simulink model "sampleModel208"  (R2021b)
settings: Solver=VariableStepAuto  StartTime=0.0  StopTime=10.0  RelTol=1e-3
undefined symbols (not defined in the file or in its folder): DiscIntNeverNeededParam, Newton, Raphson
libraries: simulink x23, slpidlib x3
settings Model: Creator=user  LastModifiedBy=user

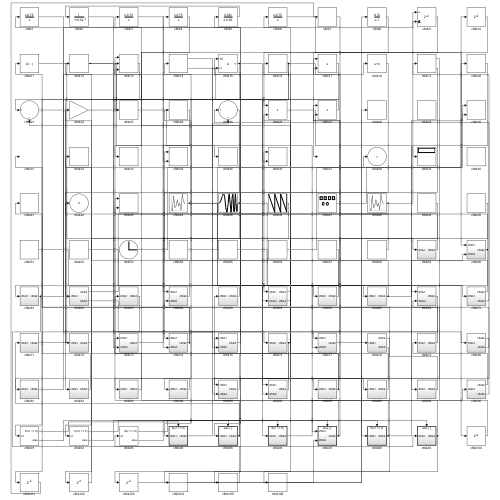
[thumbnail: Simulink's stored preview of the top-level diagram]
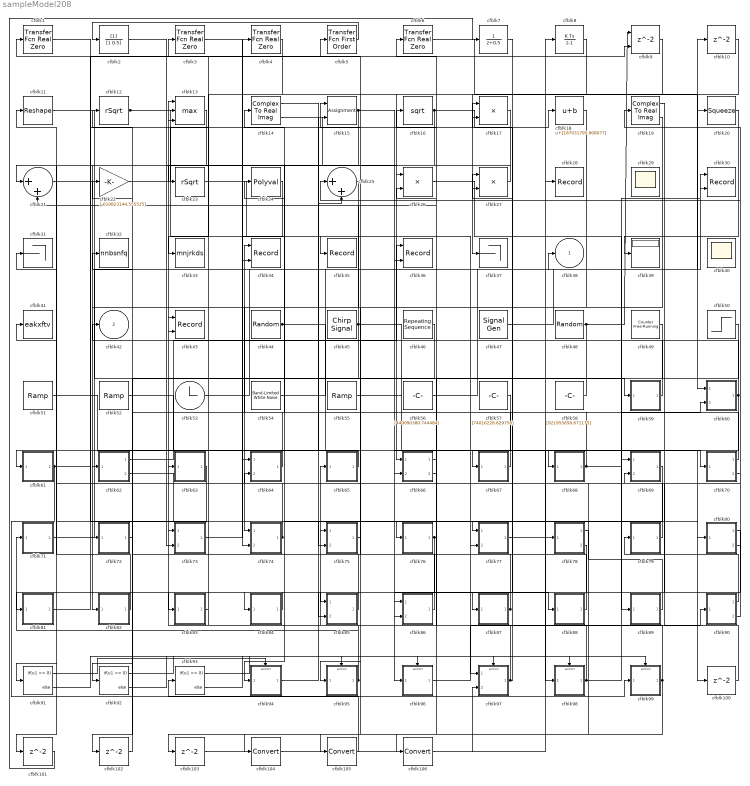
== system sampleModel208 ==
  cfblk{1,3..4,6} (4 alike) : simulink/Discrete/Transfer Fcn Real Zero  ZeroZ=0.75  ICPrevInput=0.0  DoSatur=off
      settings: SourceProductBaseCode=SL
  cfblk{10,100..103} (5 alike) : Delay  SampleTime=1
  cfblk104 : DataTypeConversion
  cfblk105 : DataTypeConversion
  cfblk106 : DataTypeConversion
  cfblk11 : Reshape
  cfblk12 : Sqrt  Operator=rSqrt  AlgorithmType=Newton-Raphson  SaturateOnIntegerOverflow=on
  cfblk13 : MinMax  Function=max  Inputs=3
  cfblk14 : ComplexToRealImag
  cfblk15 : Assignment  DiagnosticForDimensions=Warning  IndexOptions=Index vector (dialog)  Indices=1  OutputSizes=1
  cfblk16 : Sqrt  SaturateOnIntegerOverflow=on
  cfblk17 : Product
  cfblk18 : Bias  Bias=[187031795.908077]
  cfblk19 : ComplexToRealImag
  cfblk2 : DiscreteFilter  SampleTime=1
  cfblk20 : Squeeze
  cfblk21 : Sum  Inputs=|++
  cfblk22 : Gain  Gain=[-610823144.555525]
  cfblk23 : Sqrt  Operator=rSqrt  AlgorithmType=Newton-Raphson  SaturateOnIntegerOverflow=on
  cfblk24 : Polyval  Coefs=[ +2.081618890e-019, -1.441693666e-014, +4.719686976e-010, -8.536869453e-006, +1.621573104e-001, -8.087801117e+001 ]
  cfblk25 : Sum  Inputs=|++
  cfblk26 : Product
  cfblk27 : Product  Inputs=**
  cfblk28 : Record  FileSettingsInternal="{\"entries\":[{\"content\":{\"excelSettings\":{\"content\":{},\"type\":\"Streamout.ExcelSettings\"}},\"type\":\"Streamout.FileSettingStorage\",\"uuid\":\"c22ba1ce-0fcd-43a5-9d90-0db8329606c8\"}],\"packageUris\":[\"http://schema.mathworks.com/mf0/streamout_blocks/R2020a\"],\"version\":\"1.0\"}"  SignalsInternal="{\"entries\":[{\"content\":{\"signals\":[{\"content\":{\"blockPath\":[\"sampleModel208/cfblk28\"],\"channel\":[],\"dimensions\":[1],\"domain\":\"sampleModel208/cfblk28\",\"lineColor\":\"#d95319\",\"plots\":[1],\"port\":1,\"sid\":[\"\"],\"signalID\":8022,\"signalName\":\"cfblk104\"},\"type\":\"RecordBlkView.Signal\",\"uuid\":\"261dbd1d-26c2-4045-9e24-154e5f0ad3fe\"}]},\"type\":\"RecordBlkView.InputSignals\",\"uuid\":\"b79c4309-7b5a-40c4-895f-b2cc34602c3d\"}],\"packageUris\":[\"http://schema.mathworks.com/mf0/streamout_blocks/R2020a\"],\"version\":\"1.0\"}"  VisualizationBindings="{\"sparklinesplugin\":{\"info\":[{\"bindingParametersList\":[],\"subplotID\":1}]}}"
  cfblk29 : Scope
      settings: Floating=on
  cfblk30 : Record  FileSettingsInternal="{\"entries\":[{\"content\":{\"excelSettings\":{\"content\":{},\"type\":\"Streamout.ExcelSettings\"}},\"type\":\"Streamout.FileSettingStorage\",\"uuid\":\"b5dc1131-858a-47e8-ba90-4585db02b6d4\"}],\"packageUris\":[\"http://schema.mathworks.com/mf0/streamout_blocks/R2020a\"],\"version\":\"1.0\"}"  Layout=[1 1]  SignalsInternal="{\"entries\":[{\"content\":{\"signals\":[{\"content\":{\"blockPath\":[\"sampleModel208/cfblk30\"],\"channel\":[],\"dimensions\":[1],\"domain\":\"sampleModel208/cfblk30\",\"lineColor\":\"#a2142f\",\"plots\":[1],\"port\":1,\"sid\":[\"\"],\"signalID\":8026,\"signalName\":\"cfblk54\"},\"type\":\"RecordBlkView.Signal\",\"uuid\":\"3317f2e0-9c09-47a8-be30-a309801c78f4\"},{\"content\":{\"blockPath\":[\"sampleModel208/cfblk30\"],\"channel\":[],\"dimensions\":[1],\"domain\":\"sampleModel208/cfblk30\",\"lineColor\":\"#139fff\",\"plots\":[1],\"port\":2,\"sid\":[\"\"],\"signalID\":8030,\"signalName\":\"cfblk68\"},\"type\":\"RecordBlkView.Signal\",\"uuid\":\"8cfe8237-c0e8-4d48-b3ed-0524deef0457\"}]},\"type\":\"RecordBlkView.InputSignals\",\"uuid\":\"ba5baa30-43f7-4293-854a-121f9ae80c9b\"}],\"packageUris\":[\"http://schema.mathworks.com/mf0/streamout_blocks/R2020a\"],\"version\":\"1.0\"}"  VisualizationBindings="{\"xyplotplugin\":{\"info\":[{\"series\":[{\"bindingParametersList\":[{\"parameter\":\"X-Axis\",\"signalID\":8026,\"signalName\":\"cfblk54\"},{\"parameter\":\"Y-Axis\",\"signalID\":8030,\"signalName\":\"cfblk68\"}],\"seriesID\":18668}],\"subplotID\":1}]}}"  CompatibilityTag=XY
  cfblk31 : Terminator
  cfblk32 : ToWorkspace  VariableName=nnbsnfq  SaveFormat=Timeseries  SampleTime=-1
  cfblk33 : ToWorkspace  VariableName=mnjrkds  SaveFormat=Timeseries  SampleTime=-1
  cfblk34 : Record  FileSettingsInternal="{\"entries\":[{\"content\":{\"excelSettings\":{\"content\":{},\"type\":\"Streamout.ExcelSettings\"}},\"type\":\"Streamout.FileSettingStorage\",\"uuid\":\"4f32d4e9-02ed-4236-9ce3-c0bcdef04756\"}],\"packageUris\":[\"http://schema.mathworks.com/mf0/streamout_blocks/R2020a\"],\"version\":\"1.0\"}"  Layout=[1 1]  SignalsInternal="{\"entries\":[{\"content\":{\"signals\":[{\"content\":{\"blockPath\":[\"sampleModel208/cfblk34\"],\"channel\":[],\"dimensions\":[1],\"domain\":\"sampleModel208/cfblk34\",\"lineColor\":\"#a2142f\",\"plots\":[1],\"port\":1,\"sid\":[\"\"],\"signalID\":8054,\"signalName\":\"cfblk64\"},\"type\":\"RecordBlkView.Signal\",\"uuid\":\"7ea00e73-cf0b-4523-9dfb-d0665cf2003d\"},{\"content\":{\"blockPath\":[\"sampleModel208/cfblk34\"],\"channel\":[],\"dimensions\":[1],\"domain\":\"sampleModel208/cfblk34\",\"lineColor\":\"#139fff\",\"plots\":[1],\"port\":2,\"sid\":[\"\"],\"signalID\":8058,\"signalName\":\"cfblk24\"},\"type\":\"RecordBlkView.Signal\",\"uuid\":\"3ec3da29-cb72-43d4-ab85-a156e7dbbd36\"}]},\"type\":\"RecordBlkView.InputSignals\",\"uuid\":\"b859cf70-4a05-42e5-becb-aa8dfd0be4f3\"}],\"packageUris\":[\"http://schema.mathworks.com/mf0/streamout_blocks/R2020a\"],\"version\":\"1.0\"}"  VisualizationBindings="{\"xyplotplugin\":{\"info\":[{\"series\":[{\"bindingParametersList\":[{\"parameter\":\"X-Axis\",\"signalID\":8054,\"signalName\":\"cfblk64\"},{\"parameter\":\"Y-Axis\",\"signalID\":8058,\"signalName\":\"cfblk24\"}],\"seriesID\":28405}],\"subplotID\":1}]}}"  CompatibilityTag=XY
  cfblk35 : Record  FileSettingsInternal="{\"entries\":[{\"content\":{\"excelSettings\":{\"content\":{},\"type\":\"Streamout.ExcelSettings\"}},\"type\":\"Streamout.FileSettingStorage\",\"uuid\":\"4d5d1943-00c1-4ccc-bfc5-894631c5acb5\"}],\"packageUris\":[\"http://schema.mathworks.com/mf0/streamout_blocks/R2020a\"],\"version\":\"1.0\"}"  SignalsInternal="{\"entries\":[{\"content\":{\"signals\":[{\"content\":{\"blockPath\":[\"sampleModel208/cfblk35\"],\"channel\":[],\"dimensions\":[1],\"domain\":\"sampleModel208/cfblk35\",\"lineColor\":\"#77ac30\",\"plots\":[1],\"port\":1,\"sid\":[\"\"],\"signalID\":8034,\"signalName\":\"cfblk23\"},\"type\":\"RecordBlkView.Signal\",\"uuid\":\"a308330b-7e8f-4a04-a4b5-6eaafb41392d\"}]},\"type\":\"RecordBlkView.InputSignals\",\"uuid\":\"e134a712-f80f-465f-b2ee-20551d8e1273\"}],\"packageUris\":[\"http://schema.mathworks.com/mf0/streamout_blocks/R2020a\"],\"version\":\"1.0\"}"  VisualizationBindings="{\"sparklinesplugin\":{\"info\":[{\"bindingParametersList\":[],\"subplotID\":1}]}}"
  cfblk36 : Record  FileSettingsInternal="{\"entries\":[{\"content\":{\"excelSettings\":{\"content\":{},\"type\":\"Streamout.ExcelSettings\"}},\"type\":\"Streamout.FileSettingStorage\",\"uuid\":\"a0d14922-92c5-4109-8193-fc27ce21709e\"}],\"packageUris\":[\"http://schema.mathworks.com/mf0/streamout_blocks/R2020a\"],\"version\":\"1.0\"}"  Layout=[1 1]  SignalsInternal="{\"entries\":[{\"content\":{\"signals\":[{\"content\":{\"blockPath\":[\"sampleModel208/cfblk36\"],\"channel\":[],\"dimensions\":[1],\"domain\":\"sampleModel208/cfblk36\",\"lineColor\":\"#a2142f\",\"plots\":[1],\"port\":1,\"sid\":[\"\"],\"signalID\":8038,\"signalName\":\"cfblk62:1\"},\"type\":\"RecordBlkView.Signal\",\"uuid\":\"cf392b0d-73b1-445c-b980-8f3ea822809a\"},{\"content\":{\"blockPath\":[\"sampleModel208/cfblk36\"],\"channel\":[],\"dimensions\":[1],\"domain\":\"sampleModel208/cfblk36\",\"lineColor\":\"#139fff\",\"plots\":[1],\"port\":2,\"sid\":[\"\"],\"signalID\":8042,\"signalName\":\"cfblk16\"},\"type\":\"RecordBlkView.Signal\",\"uuid\":\"24cc8bd0-c2dc-4a3d-a0ab-d3c31cd0a1be\"}]},\"type\":\"RecordBlkView.InputSignals\",\"uuid\":\"8c2f2ea3-48ed-4664-b571-c4b9f4e82adb\"}],\"packageUris\":[\"http://schema.mathworks.com/mf0/streamout_blocks/R2020a\"],\"version\":\"1.0\"}"  VisualizationBindings="{\"xyplotplugin\":{\"info\":[{\"series\":[{\"bindingParametersList\":[{\"parameter\":\"X-Axis\",\"signalID\":8038,\"signalName\":\"cfblk62:1\"},{\"parameter\":\"Y-Axis\",\"signalID\":8042,\"signalName\":\"cfblk16\"}],\"seriesID\":24383}],\"subplotID\":1}]}}"  CompatibilityTag=XY
  cfblk37 : Terminator
  cfblk39 : Display
  cfblk40 : Scope
      settings: Floating=on
  cfblk41 : ToWorkspace  VariableName=eakxftv  SaveFormat=Timeseries  SampleTime=-1
  cfblk43 : Record  FileSettingsInternal="{\"entries\":[{\"content\":{\"excelSettings\":{\"content\":{},\"type\":\"Streamout.ExcelSettings\"}},\"type\":\"Streamout.FileSettingStorage\",\"uuid\":\"00404128-d092-4654-98f3-0c769e6ce3be\"}],\"packageUris\":[\"http://schema.mathworks.com/mf0/streamout_blocks/R2020a\"],\"version\":\"1.0\"}"  Layout=[1 1]  SignalsInternal="{\"entries\":[{\"content\":{\"signals\":[{\"content\":{\"blockPath\":[\"sampleModel208/cfblk43\"],\"channel\":[],\"dimensions\":[1],\"domain\":\"sampleModel208/cfblk43\",\"lineColor\":\"#a2142f\",\"plots\":[1],\"port\":1,\"sid\":[\"\"],\"signalID\":8046,\"signalName\":\"cfblk79\"},\"type\":\"RecordBlkView.Signal\",\"uuid\":\"ce2b062f-3cfe-4973-a794-e20ce7e23f9b\"},{\"content\":{\"blockPath\":[\"sampleModel208/cfblk43\"],\"channel\":[],\"dimensions\":[1],\"domain\":\"sampleModel208/cfblk43\",\"lineColor\":\"#139fff\",\"plots\":[1],\"port\":2,\"sid\":[\"\"],\"signalID\":8050,\"signalName\":\"cfblk48\"},\"type\":\"RecordBlkView.Signal\",\"uuid\":\"da814807-78ce-423b-937a-9547f0faf18a\"}]},\"type\":\"RecordBlkView.InputSignals\",\"uuid\":\"e4b74333-ca83-42be-81e0-1eb5d34b8ec7\"}],\"packageUris\":[\"http://schema.mathworks.com/mf0/streamout_blocks/R2020a\"],\"version\":\"1.0\"}"  VisualizationBindings="{\"xyplotplugin\":{\"info\":[{\"series\":[{\"bindingParametersList\":[{\"parameter\":\"X-Axis\",\"signalID\":8046,\"signalName\":\"cfblk79\"},{\"parameter\":\"Y-Axis\",\"signalID\":8050,\"signalName\":\"cfblk48\"}],\"seriesID\":25686}],\"subplotID\":1}]}}"  CompatibilityTag=XY
  cfblk44 : UniformRandomNumber  Minimum=[-5209162267.996864]  Maximum=[7486341106.977611]  Seed=[64925626.000000]  SampleTime=0.1
  cfblk45 : simulink/Sources/Chirp Signal  f1=[-755698620.571404]  T=[-833933526.641706]  f2=[267223703.943291]
  cfblk46 : simulink/Sources/Repeating Sequence  rep_seq_t=[0 2]  rep_seq_y=[919874426.508816, 363568850.149377]
  cfblk47 : SignalGenerator  WaveForm=square  Amplitude=[217272616.194499]
  cfblk48 : UniformRandomNumber  Minimum=[-5223909817.198769]  Maximum=[5188022340.697088]  Seed=[56413417.000000]  SampleTime=0.1
  cfblk49 : simulink/Sources/Counter Free-Running  NumBits=[41.000000]  tsamp=-1
  cfblk5 : simulink/Discrete/Transfer Fcn First Order  PoleZ=0.95  ICPrevOutput=0.0  DoSatur=off
  cfblk50 : Step  Time=[15.000000]  Before=[292405392.362123]  After=[-377924494.241017]  SampleTime=0
  cfblk51 : simulink/Sources/Ramp  slope=[5467.724857]  start=[19.133778]  InitialOutput=[29297.594376]
  cfblk52 : simulink/Sources/Ramp  slope=[706.412132]  start=[13.023382]  InitialOutput=[-774712.176920]
  cfblk53 : Clock
  cfblk54 : simulink/Sources/Band-Limited White Noise  Cov=[6259669263.783980]  Ts=0.1  seed=[9291998557.000000]
  cfblk55 : simulink/Sources/Ramp  slope=[-6341.235505]  start=[31.577316]  InitialOutput=[-676904.104674]
  cfblk56 : Constant  Value=[440090380.744484]  SampleTime=1
  cfblk57 : Constant  Value=[74016228.829758]  SampleTime=1
  cfblk58 : Constant  Value=[921955858.671175]  SampleTime=1
  cfblk59 : Subsystem
  cfblk60 : Subsystem
  cfblk61 : Subsystem
  cfblk62 : Subsystem
  cfblk63 : Subsystem
  cfblk64 : Subsystem
  cfblk65 : Subsystem
  cfblk66 : Subsystem
  cfblk67 : Subsystem
  cfblk68 : Subsystem
  cfblk69 : Subsystem
  cfblk7 : DiscreteTransferFcn  SampleTime=1
  cfblk70 : Subsystem
  cfblk71 : Subsystem
  cfblk72 : Subsystem
  cfblk73 : Subsystem
  cfblk74 : Subsystem
  cfblk75 : Subsystem
  cfblk76 : Subsystem
  cfblk77 : Subsystem
  cfblk78 : Subsystem
  cfblk79 : Subsystem
  cfblk8 : DiscreteIntegrator  ICPrevOutput=DiscIntNeverNeededParam  ICPrevScaledInput=DiscIntNeverNeededParam
  cfblk80 : Subsystem
  cfblk81 : Subsystem
  cfblk82 : Subsystem
  cfblk83 : Subsystem
  cfblk84 : Subsystem
  cfblk85 : Subsystem
  cfblk86 : Subsystem
  cfblk87 : Subsystem
  cfblk88 : Subsystem
  cfblk89 : Subsystem
  cfblk9 : Delay  ShowEnablePort=on  SampleTime=1
      settings: InputPortMap=u0,e6
  cfblk90 : Subsystem
  cfblk91 : If  IfExpression=u1 >= 0  SampleTime=1
  cfblk92 : If  IfExpression=u1 >= 0  SampleTime=1
  cfblk93 : If  IfExpression=u1 >= 0  SampleTime=1
  cfblk94 : Subsystem  TreatAsAtomicUnit=on
  cfblk95 : Subsystem  TreatAsAtomicUnit=on
  cfblk96 : Subsystem  TreatAsAtomicUnit=on
  cfblk97 : Subsystem  TreatAsAtomicUnit=on
  cfblk98 : Subsystem  TreatAsAtomicUnit=on
  cfblk99 : Subsystem  TreatAsAtomicUnit=on
  cfblk38 : Outport
  cfblk42 : Outport  Port=2
  wires:
  cfblk64/1(cfblk2) -> cfblk34/1
  cfblk97/1(cfblk2) -> cfblk65/1(cfblk1), cfblk27/2
  cfblk88/1(cfblk2) -> cfblk75/1(cfblk1)
  cfblk9/1 -> cfblk66/1(cfblk1)
  cfblk90/1(cfblk2) -> cfblk79/1(cfblk1)
  cfblk13/1 -> cfblk82/1(cfblk1)
  cfblk89/1(cfblk2) -> cfblk1/1
  cfblk73/1(cfblk2) -> cfblk4/1
  cfblk95/1(cfblk2) -> cfblk71/1(cfblk1), cfblk73/1(cfblk1)
  cfblk16/1 -> cfblk18/1, cfblk36/2, cfblk73/2(cfblk5)
  cfblk58/1 -> cfblk14/1
  cfblk85/1(cfblk2) -> cfblk13/1
  cfblk90/2(cfblk5) -> cfblk25/1
  cfblk54/1 -> cfblk30/1
  cfblk10/1 -> cfblk37/1
  cfblk87/1(cfblk2) -> cfblk15/1, cfblk26/2
  cfblk61/1(cfblk2) -> cfblk99/1(cfblk1), cfblk13/3
  cfblk56/1 -> cfblk20/1
  cfblk18/1 -> cfblk95/1(cfblk1)
  cfblk83/1(cfblk2) -> cfblk3/1
  cfblk48/1 -> cfblk9/1, cfblk43/2
  cfblk65/1(cfblk2) -> cfblk61/1(cfblk1)
  cfblk23/1 -> cfblk35/1
  cfblk8/1 -> cfblk33/1
  cfblk12/1 -> cfblk97/1(cfblk1), cfblk76/1(cfblk1)
  cfblk51/1 -> cfblk68/1(cfblk1)
  cfblk27/1 -> cfblk21/1
  cfblk74/1(cfblk2) -> cfblk31/1, cfblk41/1
  cfblk79/1(cfblk2) -> cfblk43/1
  cfblk98/1(cfblk2) -> cfblk16/1, cfblk60/2(cfblk5)
  cfblk7/1 -> cfblk87/1(cfblk1)
  cfblk14/1 -> cfblk70/1(cfblk1)
  cfblk2/1 -> cfblk26/1
  cfblk71/1(cfblk2) -> cfblk38/1
  cfblk19/1 -> cfblk85/1(cfblk1)
  cfblk99/1(cfblk2) -> cfblk63/1(cfblk1), cfblk103/1
  cfblk84/1(cfblk2) -> cfblk81/1(cfblk1)
  cfblk52/1 -> cfblk80/1(cfblk1)
  cfblk81/1(cfblk2) -> cfblk9/2
  cfblk67/1(cfblk2) -> cfblk24/1
  cfblk82/1(cfblk2) -> cfblk11/1
  cfblk20/1 -> cfblk39/1
  cfblk19/2 -> cfblk74/1(cfblk1)
  cfblk44/1 -> cfblk89/1(cfblk1), cfblk96/1(cfblk1)
  cfblk75/1(cfblk2) -> cfblk5/1
  cfblk14/2 -> cfblk86/1(cfblk1)
  cfblk22/1 -> cfblk17/1
  cfblk94/1(cfblk2) -> cfblk25/2
  cfblk96/1(cfblk2) -> cfblk90/1(cfblk1)
  cfblk3/1 -> cfblk64/1(cfblk1)
  cfblk11/1 -> cfblk59/1(cfblk1)
  cfblk80/1(cfblk2) -> cfblk83/1(cfblk1)
  cfblk25/1 -> cfblk72/1(cfblk1)
  cfblk47/1 -> cfblk10/1
  cfblk5/1 -> cfblk2/1
  cfblk53/1 -> cfblk15/2
  cfblk24/1 -> cfblk34/2
  cfblk21/1 -> cfblk62/1(cfblk1)
  cfblk45/1 -> cfblk74/2(cfblk3), cfblk77/2(cfblk5), cfblk13/2
  cfblk6/1 -> cfblk60/1(cfblk1)
  cfblk76/1(cfblk2) -> cfblk6/1, cfblk86/2(cfblk5)
  cfblk63/1(cfblk2) -> cfblk91/1
  cfblk86/1(cfblk2) -> cfblk32/1
  cfblk55/1 -> cfblk98/1(cfblk1)
  cfblk66/1(cfblk2) -> cfblk85/2(cfblk4)
  cfblk15/1 -> cfblk88/1(cfblk1), cfblk101/1
  cfblk80/2(cfblk4) -> cfblk64/2(cfblk5)
  cfblk26/1 -> cfblk69/1(cfblk1)
  cfblk66/2(cfblk4) -> cfblk21/2
  cfblk77/1(cfblk2) -> cfblk8/1
  cfblk60/1(cfblk2) -> cfblk27/1, cfblk66/2(cfblk3)
  cfblk62/1(cfblk2) -> cfblk36/1
  cfblk59/1(cfblk2) -> cfblk42/1
  cfblk4/1 -> cfblk23/1
  cfblk17/1 -> cfblk94/1(cfblk1)
  cfblk46/1 -> cfblk92/1
  cfblk1/1 -> cfblk75/2(cfblk5)
  cfblk69/1(cfblk2) -> cfblk84/1(cfblk1)
  cfblk70/1(cfblk2) -> cfblk22/1
  cfblk57/1 -> cfblk67/1(cfblk1)
  cfblk70/2(cfblk3) -> cfblk19/1
  cfblk68/1(cfblk2) -> cfblk30/2, cfblk17/2
  cfblk50/1 -> cfblk77/1(cfblk1)
  cfblk91/1 -> cfblk94/Action
  cfblk91/2 -> cfblk95/Action
  cfblk92/1 -> cfblk96/Action
  cfblk92/2 -> cfblk97/Action
  cfblk93/1 -> cfblk98/Action
  cfblk93/2 -> cfblk99/Action
  cfblk62/2(cfblk3) -> cfblk100/1
  cfblk100/1 -> cfblk69/2(cfblk3)
  cfblk101/1 -> cfblk7/1
  cfblk72/1(cfblk2) -> cfblk102/1
  cfblk102/1 -> cfblk12/1
  cfblk103/1 -> cfblk97/2(cfblk4)
  cfblk78/1(cfblk2) -> cfblk104/1
  cfblk104/1 -> cfblk28/1
  cfblk78/2(cfblk3) -> cfblk105/1
  cfblk105/1 -> cfblk93/1
  cfblk49/1 -> cfblk106/1
  cfblk106/1 -> cfblk78/1(cfblk1)

== system sampleModel208/cfblk59 ==
  cfblk1 : Inport
  cfblk3 : DiscreteIntegrator  ICPrevOutput=DiscIntNeverNeededParam  ICPrevScaledInput=DiscIntNeverNeededParam
  cfblk2 : Outport
  wires:
  cfblk1/1 -> cfblk2/1, cfblk3/1

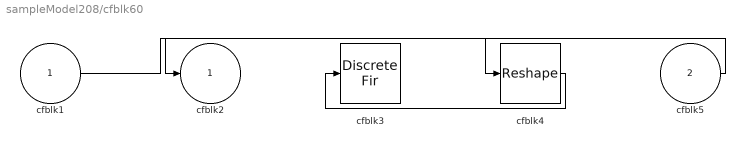
== system sampleModel208/cfblk60 ==
  cfblk1 : Inport
  cfblk5 : Inport  Port=2
  cfblk3 : DiscreteFir  SampleTime=1
  cfblk4 : Reshape
  cfblk2 : Outport
  wires:
  cfblk5/1 -> cfblk2/1
  cfblk4/1 -> cfblk3/1
  cfblk1/1 -> cfblk4/1

== system sampleModel208/cfblk61 ==
  cfblk1 : Inport
  cfblk3 : simulink/Discrete/Difference  ICPrevInput=0.0  OutMin=[]  OutMax=[]  OutDataTypeStr=Inherit: Inherit via back propagation  OutDataType=fixdt(1, 16)  OutScaling=2^-10  DoSatur=off
  cfblk4 : ComplexToRealImag
  cfblk2 : Outport
  wires:
  cfblk1/1 -> cfblk3/1
  cfblk4/1 -> cfblk2/1
  cfblk3/1 -> cfblk4/1

== system sampleModel208/cfblk62 ==
  cfblk1 : Inport
  cfblk2 : Outport
  cfblk3 : Outport  Port=2
  wires:
  cfblk1/1 -> cfblk2/1, cfblk3/1

== system sampleModel208/cfblk63 ==
  cfblk1 : Inport
  cfblk3 : Polyval  Coefs=[ +2.081618890e-019, -1.441693666e-014, +4.719686976e-010, -8.536869453e-006, +1.621573104e-001, -8.087801117e+001 ]
  cfblk2 : Outport
  wires:
  cfblk1/1 -> cfblk3/1
  cfblk3/1 -> cfblk2/1

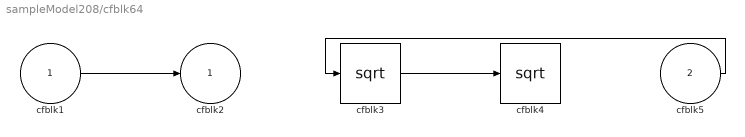
== system sampleModel208/cfblk64 ==
  cfblk1 : Inport
  cfblk5 : Inport  Port=2
  cfblk3 : Sqrt  SaturateOnIntegerOverflow=on
  cfblk4 : Sqrt  SaturateOnIntegerOverflow=on
  cfblk2 : Outport
  wires:
  cfblk1/1 -> cfblk2/1
  cfblk5/1 -> cfblk3/1
  cfblk3/1 -> cfblk4/1

== system sampleModel208/cfblk65 ==
  cfblk1 : Inport
  cfblk3 : Constant  Value=[606104915.024978]  SampleTime=1
  cfblk2 : Outport
  wires:
  cfblk1/1 -> cfblk2/1

== system sampleModel208/cfblk66 ==
  cfblk1 : Inport
  cfblk3 : Inport  Port=2
  cfblk2 : Outport
  cfblk4 : Outport  Port=2
  wires:
  cfblk3/1 -> cfblk4/1
  cfblk1/1 -> cfblk2/1

== system sampleModel208/cfblk67 ==
  cfblk1 : Inport
  cfblk3 : Delay  SampleTime=1
  cfblk4 : slpidlib/PID Controller  Controller=PID  Form=Parallel  TimeDomain=Discrete-time  UseExternalTs=off  SampleTime=1  IntegratorMethod=Forward Euler  FilterMethod=Forward Euler  ControllerParametersSource=internal  P=1  I=1  D=0  UseFilter=on  N=100  TunerSelectOption=Transfer Function Based (PID Tuner App)  InitialConditionSource=internal  InitialConditionForIntegrator=0  InitialConditionForFilter=0  DifferentiatorICPrevScaledInput=0  ExternalReset=none  TrackingMode=off  Kt=1  LimitOutput=off  SatLimitsSource=internal  UpperSaturationLimit=inf  LowerSaturationLimit=-inf  LinearizeAsGain=off  AntiWindupMode=none  Kb=1  POutMin=[]  POutMax=[]  IOutMin=[]  IOutMax=[]  DOutMin=[]  DOutMax=[]  NOutMin=[]  NOutMax=[]  SumOutMin=[]  SumOutMax=[]  SaturationOutMin=[]  SaturationOutMax=[]  PParamMin=[]  PParamMax=[]  IParamMin=[]  IParamMax=[]  DParamMin=[]  DParamMax=[]  NParamMin=[]  NParamMax=[]  KbParamMin=[]  KbParamMax=[]  KtParamMin=[]  KtParamMax=[]  KbOutMin=[]  KbOutMax=[]  KtOutMin=[]  KtOutMax=[]  IntegratorOutMin=[]  IntegratorOutMax=[]  FilterOutMin=[]  FilterOutMax=[]  SumI1OutMin=[]  SumI1OutMax=[]  SumI2OutMin=[]  SumI2OutMax=[]  SumI3OutMin=[]  SumI3OutMax=[]  SumI4OutMin=[]  SumI4OutMax=[]  SumDOutMin=[]  SumDOutMax=[]  DifferentiatorOutMin=[]  DifferentiatorOutMax=[]  FilterDiffOutCoefMin=[]  FilterDiffOutCoefMax=[]  ReciprocalOutMin=[]  ReciprocalOutMax=[]  SumDenOutMin=[]  SumDenOutMax=[]  SumNumOutMin=[]  SumNumOutMax=[]  DivideOutMin=[]  DivideOutMax=[]  UdiffTsProdOutMin=[]  UdiffTsProdOutMax=[]  NTsProdOutMin=[]  NTsProdOutMax=[]  UintegralTsProdOutMin=[]  UintegralTsProdOutMax=[]  UngainTsProdOutMin=[]  UngainTsProdOutMax=[]  IntegratorContinuousStateAttributes=''  IntegratorStateMustResolveToSignalObject=off  IntegratorRTWStateStorageClass=Auto  FilterContinuousStateAttributes=''  FilterStateMustResolveToSignalObject=off  FilterRTWStateStorageClass=Auto  ParallelPVariant=InternalParameters  IdealPVariant=Disabled  IVariant=InternalParameters  DVariant=InternalParameters  IntegratorVariant=Discrete  SatVariant=Disabled  AWVariant=Passthrough  PCopyVariant=Disabled  TRVariant=Disabled  FdbkBlocksVariant=Forward  IdealPFdbkVariant=Disabled  SatFdbkVariant=Disabled  DerivativeFilterVariant=ForwardEulerFilter  NVariant=InternalParameters  NCopyVariant=Disabled  FilterICVariant=InternalICsFilter  IntegratorICVariant=InternalICs  ExternalResetVariant=Disabled  TRSumVariant=Passthrough  SumFdbkVariant=Disabled  SumVariant=Sum_PID  TsampFilterVariant=InternalTs  TsampNgainVariant=Passthrough  TsampIntegralVariant=Passthrough  ExternalSaturationOutDataTypeStr=Inherit: Same as second input
  cfblk2 : Outport
  wires:
  cfblk1/1 -> cfblk3/1
  cfblk4/1 -> cfblk2/1
  cfblk3/1 -> cfblk4/1

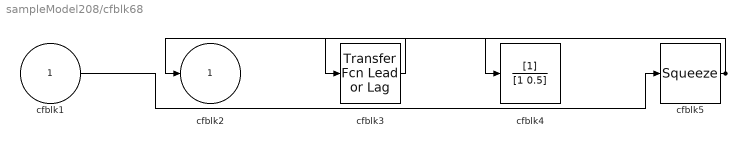
== system sampleModel208/cfblk68 ==
  cfblk1 : Inport
  cfblk3 : simulink/Discrete/Transfer Fcn Lead or Lag  PoleZ=0.95  ZeroZ=0.75  ICPrevOutput=0.0  ICPrevInput=0.0  DoSatur=off
      settings: SourceProductBaseCode=SL
  cfblk4 : DiscreteFilter  SampleTime=1
  cfblk5 : Squeeze
  cfblk2 : Outport
  wires:
  cfblk3/1 -> cfblk2/1
  cfblk1/1 -> cfblk5/1
  cfblk5/1 -> cfblk3/1, cfblk4/1

== system sampleModel208/cfblk69 ==
  cfblk1 : Inport
  cfblk3 : Inport  Port=2
  cfblk2 : Outport
  wires:
  cfblk1/1 -> cfblk2/1

== system sampleModel208/cfblk70 ==
  cfblk1 : Inport
  cfblk2 : Outport
  cfblk3 : Outport  Port=2
  wires:
  cfblk1/1 -> cfblk3/1, cfblk2/1

== system sampleModel208/cfblk71 ==
  cfblk1 : Inport
  cfblk3 : Math  Operator=conj  SaturateOnIntegerOverflow=on
  cfblk2 : Outport
  wires:
  cfblk3/1 -> cfblk2/1
  cfblk1/1 -> cfblk3/1

== system sampleModel208/cfblk72 ==
  cfblk1 : Inport
  cfblk3 : Delay  ShowEnablePort=on  SampleTime=1
      settings: InputPortMap=u0,e6
  cfblk2 : Outport
  wires:
  cfblk3/1 -> cfblk2/1
  cfblk1/1 -> cfblk3/1, cfblk3/2

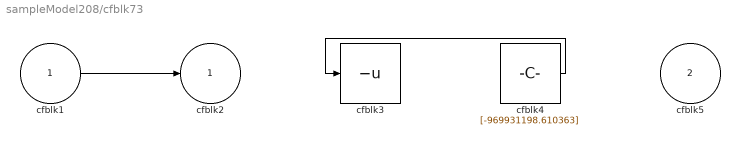
== system sampleModel208/cfblk73 ==
  cfblk1 : Inport
  cfblk5 : Inport  Port=2
  cfblk3 : UnaryMinus
  cfblk4 : Constant  Value=[-969931198.610363]  SampleTime=1
  cfblk2 : Outport
  wires:
  cfblk1/1 -> cfblk2/1
  cfblk4/1 -> cfblk3/1

== system sampleModel208/cfblk74 ==
  cfblk1 : Inport
  cfblk3 : Inport  Port=2
  cfblk2 : Outport
  wires:
  cfblk3/1 -> cfblk2/1

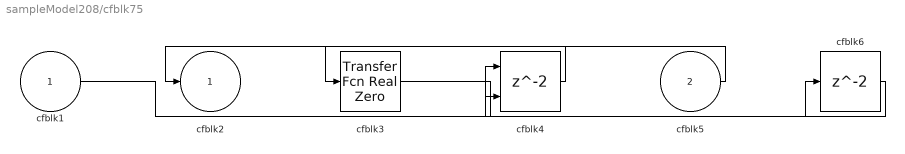
== system sampleModel208/cfblk75 ==
  cfblk1 : Inport
  cfblk5 : Inport  Port=2
  cfblk3 : simulink/Discrete/Transfer Fcn Real Zero  ZeroZ=0.75  ICPrevInput=0.0  DoSatur=off
      settings: SourceProductBaseCode=SL
  cfblk4 : Delay  ShowEnablePort=on  SampleTime=1
      settings: InputPortMap=u0,e6
  cfblk6 : Delay  SampleTime=1
  cfblk2 : Outport
  wires:
  cfblk5/1 -> cfblk2/1
  cfblk1/1 -> cfblk4/1
  cfblk4/1 -> cfblk3/1
  cfblk3/1 -> cfblk6/1
  cfblk6/1 -> cfblk4/2

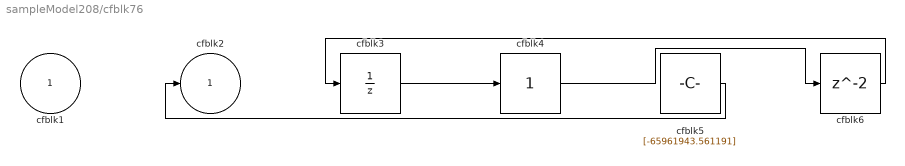
== system sampleModel208/cfblk76 ==
  cfblk1 : Inport
  cfblk3 : UnitDelay  HasFrameUpgradeWarning=on
  cfblk4 : simulink/Math Operations/Slider Gain  gain=1  low=0  high=2
  cfblk5 : Constant  Value=[-65961943.561191]  SampleTime=1
  cfblk6 : Delay  SampleTime=1
  cfblk2 : Outport
  wires:
  cfblk3/1 -> cfblk4/1
  cfblk5/1 -> cfblk2/1
  cfblk4/1 -> cfblk6/1
  cfblk6/1 -> cfblk3/1

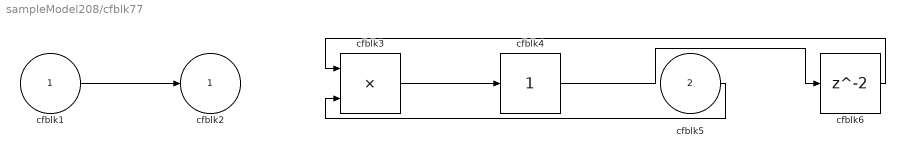
== system sampleModel208/cfblk77 ==
  cfblk1 : Inport
  cfblk5 : Inport  Port=2
  cfblk3 : Product
  cfblk4 : simulink/Math Operations/Slider Gain  gain=1  low=0  high=2
  cfblk6 : Delay  SampleTime=1
  cfblk2 : Outport
  wires:
  cfblk1/1 -> cfblk2/1
  cfblk3/1 -> cfblk4/1
  cfblk5/1 -> cfblk3/2
  cfblk4/1 -> cfblk6/1
  cfblk6/1 -> cfblk3/1

== system sampleModel208/cfblk78 ==
  cfblk1 : Inport
  cfblk2 : Outport
  cfblk3 : Outport  Port=2
  wires:
  cfblk1/1 -> cfblk2/1, cfblk3/1

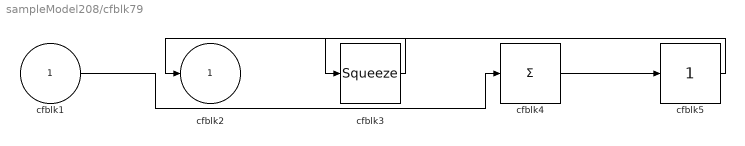
== system sampleModel208/cfblk79 ==
  cfblk1 : Inport
  cfblk3 : Squeeze
  cfblk4 : Sum  Inputs=+
  cfblk5 : simulink/Math Operations/Slider Gain  gain=1  low=0  high=2
  cfblk2 : Outport
  wires:
  cfblk4/1 -> cfblk5/1
  cfblk3/1 -> cfblk2/1
  cfblk1/1 -> cfblk4/1
  cfblk5/1 -> cfblk3/1

== system sampleModel208/cfblk80 ==
  cfblk1 : Inport
  cfblk3 : Constant  Value=[142919699.194080]  SampleTime=1
  cfblk2 : Outport
  cfblk4 : Outport  Port=2
  wires:
  cfblk1/1 -> cfblk2/1
  cfblk3/1 -> cfblk4/1

== system sampleModel208/cfblk81 ==
  cfblk1 : Inport
  cfblk3 : Sum  Inputs=|++
  cfblk2 : Outport
  wires:
  cfblk1/1 -> cfblk3/1, cfblk3/2
  cfblk3/1 -> cfblk2/1

== system sampleModel208/cfblk82 ==
  cfblk1 : Inport
  cfblk3 : Product  Inputs=**
  cfblk2 : Outport
  wires:
  cfblk1/1 -> cfblk3/1, cfblk3/2
  cfblk3/1 -> cfblk2/1

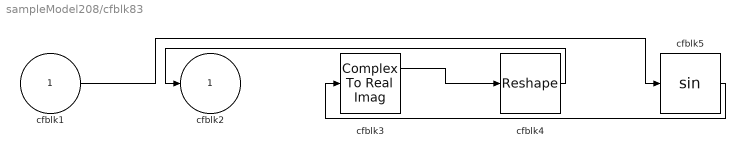
== system sampleModel208/cfblk83 ==
  cfblk1 : Inport
  cfblk3 : ComplexToRealImag
  cfblk4 : Reshape
  cfblk5 : Trigonometry
  cfblk2 : Outport
  wires:
  cfblk4/1 -> cfblk2/1
  cfblk5/1 -> cfblk3/1
  cfblk1/1 -> cfblk5/1
  cfblk3/1 -> cfblk4/1

== system sampleModel208/cfblk84 ==
  cfblk1 : Inport
  cfblk3 : simulink/Discrete/Difference  ICPrevInput=0.0  OutMin=[]  OutMax=[]  OutDataTypeStr=Inherit: Inherit via back propagation  OutDataType=fixdt(1, 16)  OutScaling=2^-10  DoSatur=off
  cfblk4 : Reshape
  cfblk2 : Outport
  wires:
  cfblk1/1 -> cfblk4/1
  cfblk4/1 -> cfblk3/1
  cfblk3/1 -> cfblk2/1

== system sampleModel208/cfblk85 ==
  cfblk1 : Inport
  cfblk4 : Inport  Port=2
  cfblk3 : Constant  Value=[587237413.607553]  SampleTime=1
  cfblk2 : Outport
  wires:
  cfblk3/1 -> cfblk2/1

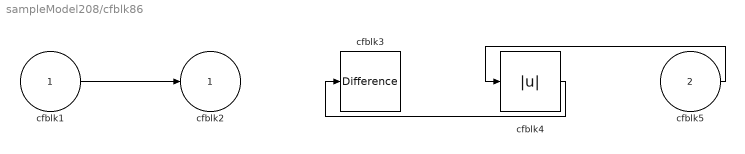
== system sampleModel208/cfblk86 ==
  cfblk1 : Inport
  cfblk5 : Inport  Port=2
  cfblk3 : simulink/Discrete/Difference  ICPrevInput=0.0  OutMin=[]  OutMax=[]  OutDataTypeStr=Inherit: Inherit via back propagation  OutDataType=fixdt(1, 16)  OutScaling=2^-10  DoSatur=off
  cfblk4 : Abs
  cfblk2 : Outport
  wires:
  cfblk1/1 -> cfblk2/1
  cfblk5/1 -> cfblk4/1
  cfblk4/1 -> cfblk3/1

== system sampleModel208/cfblk87 ==
  cfblk1 : Inport
  cfblk3 : simulink/Discrete/Transfer Fcn Real Zero  ZeroZ=0.75  ICPrevInput=0.0  DoSatur=off
      settings: SourceProductBaseCode=SL
  cfblk2 : Outport
  wires:
  cfblk1/1 -> cfblk3/1
  cfblk3/1 -> cfblk2/1

== system sampleModel208/cfblk88 ==
  cfblk1 : Inport
  cfblk3 : ComplexToMagnitudeAngle
  cfblk4 : Sin  TimeSource=Use external signal  SampleTime=0
  cfblk2 : Outport
  wires:
  cfblk4/1 -> cfblk3/1
  cfblk1/1 -> cfblk4/1
  cfblk3/1 -> cfblk2/1

== system sampleModel208/cfblk89 ==
  cfblk1 : Inport
  cfblk3 : slpidlib/PID Controller  Controller=PID  Form=Parallel  TimeDomain=Discrete-time  UseExternalTs=off  SampleTime=1  IntegratorMethod=Forward Euler  FilterMethod=Forward Euler  ControllerParametersSource=internal  P=1  I=1  D=0  UseFilter=on  N=100  TunerSelectOption=Transfer Function Based (PID Tuner App)  InitialConditionSource=internal  InitialConditionForIntegrator=0  InitialConditionForFilter=0  DifferentiatorICPrevScaledInput=0  ExternalReset=none  TrackingMode=off  Kt=1  LimitOutput=off  SatLimitsSource=internal  UpperSaturationLimit=inf  LowerSaturationLimit=-inf  LinearizeAsGain=off  AntiWindupMode=none  Kb=1  POutMin=[]  POutMax=[]  IOutMin=[]  IOutMax=[]  DOutMin=[]  DOutMax=[]  NOutMin=[]  NOutMax=[]  SumOutMin=[]  SumOutMax=[]  SaturationOutMin=[]  SaturationOutMax=[]  PParamMin=[]  PParamMax=[]  IParamMin=[]  IParamMax=[]  DParamMin=[]  DParamMax=[]  NParamMin=[]  NParamMax=[]  KbParamMin=[]  KbParamMax=[]  KtParamMin=[]  KtParamMax=[]  KbOutMin=[]  KbOutMax=[]  KtOutMin=[]  KtOutMax=[]  IntegratorOutMin=[]  IntegratorOutMax=[]  FilterOutMin=[]  FilterOutMax=[]  SumI1OutMin=[]  SumI1OutMax=[]  SumI2OutMin=[]  SumI2OutMax=[]  SumI3OutMin=[]  SumI3OutMax=[]  SumI4OutMin=[]  SumI4OutMax=[]  SumDOutMin=[]  SumDOutMax=[]  DifferentiatorOutMin=[]  DifferentiatorOutMax=[]  FilterDiffOutCoefMin=[]  FilterDiffOutCoefMax=[]  ReciprocalOutMin=[]  ReciprocalOutMax=[]  SumDenOutMin=[]  SumDenOutMax=[]  SumNumOutMin=[]  SumNumOutMax=[]  DivideOutMin=[]  DivideOutMax=[]  UdiffTsProdOutMin=[]  UdiffTsProdOutMax=[]  NTsProdOutMin=[]  NTsProdOutMax=[]  UintegralTsProdOutMin=[]  UintegralTsProdOutMax=[]  UngainTsProdOutMin=[]  UngainTsProdOutMax=[]  IntegratorContinuousStateAttributes=''  IntegratorStateMustResolveToSignalObject=off  IntegratorRTWStateStorageClass=Auto  FilterContinuousStateAttributes=''  FilterStateMustResolveToSignalObject=off  FilterRTWStateStorageClass=Auto  ParallelPVariant=InternalParameters  IdealPVariant=Disabled  IVariant=InternalParameters  DVariant=InternalParameters  IntegratorVariant=Discrete  SatVariant=Disabled  AWVariant=Passthrough  PCopyVariant=Disabled  TRVariant=Disabled  FdbkBlocksVariant=Forward  IdealPFdbkVariant=Disabled  SatFdbkVariant=Disabled  DerivativeFilterVariant=ForwardEulerFilter  NVariant=InternalParameters  NCopyVariant=Disabled  FilterICVariant=InternalICsFilter  IntegratorICVariant=InternalICs  ExternalResetVariant=Disabled  TRSumVariant=Passthrough  SumFdbkVariant=Disabled  SumVariant=Sum_PID  TsampFilterVariant=InternalTs  TsampNgainVariant=Passthrough  TsampIntegralVariant=Passthrough  ExternalSaturationOutDataTypeStr=Inherit: Same as second input
  cfblk2 : Outport
  wires:
  cfblk3/1 -> cfblk2/1
  cfblk1/1 -> cfblk3/1

== system sampleModel208/cfblk90 ==
  cfblk1 : Inport
  cfblk3 : simulink/Discrete/Transfer Fcn First Order  PoleZ=0.95  ICPrevOutput=0.0  DoSatur=off
  cfblk4 : Reshape
  cfblk2 : Outport
  cfblk5 : Outport  Port=2
  wires:
  cfblk3/1 -> cfblk2/1, cfblk4/1
  cfblk1/1 -> cfblk3/1
  cfblk4/1 -> cfblk5/1

== system sampleModel208/cfblk94 ==
  cfblk1 : Inport
  Action Port : ActionPort  ActionPortLabel=if(u1 >= 0)
  cfblk3 : slpidlib/PID Controller  Controller=PID  Form=Parallel  TimeDomain=Discrete-time  UseExternalTs=off  SampleTime=-1  IntegratorMethod=Forward Euler  FilterMethod=Forward Euler  ControllerParametersSource=internal  P=1  I=1  D=0  UseFilter=on  N=100  TunerSelectOption=Transfer Function Based (PID Tuner App)  InitialConditionSource=internal  InitialConditionForIntegrator=0  InitialConditionForFilter=0  DifferentiatorICPrevScaledInput=0  ExternalReset=none  TrackingMode=off  Kt=1  LimitOutput=off  SatLimitsSource=internal  UpperSaturationLimit=inf  LowerSaturationLimit=-inf  LinearizeAsGain=off  AntiWindupMode=none  Kb=1  POutMin=[]  POutMax=[]  IOutMin=[]  IOutMax=[]  DOutMin=[]  DOutMax=[]  NOutMin=[]  NOutMax=[]  SumOutMin=[]  SumOutMax=[]  SaturationOutMin=[]  SaturationOutMax=[]  PParamMin=[]  PParamMax=[]  IParamMin=[]  IParamMax=[]  DParamMin=[]  DParamMax=[]  NParamMin=[]  NParamMax=[]  KbParamMin=[]  KbParamMax=[]  KtParamMin=[]  KtParamMax=[]  KbOutMin=[]  KbOutMax=[]  KtOutMin=[]  KtOutMax=[]  IntegratorOutMin=[]  IntegratorOutMax=[]  FilterOutMin=[]  FilterOutMax=[]  SumI1OutMin=[]  SumI1OutMax=[]  SumI2OutMin=[]  SumI2OutMax=[]  SumI3OutMin=[]  SumI3OutMax=[]  SumI4OutMin=[]  SumI4OutMax=[]  SumDOutMin=[]  SumDOutMax=[]  DifferentiatorOutMin=[]  DifferentiatorOutMax=[]  FilterDiffOutCoefMin=[]  FilterDiffOutCoefMax=[]  ReciprocalOutMin=[]  ReciprocalOutMax=[]  SumDenOutMin=[]  SumDenOutMax=[]  SumNumOutMin=[]  SumNumOutMax=[]  DivideOutMin=[]  DivideOutMax=[]  UdiffTsProdOutMin=[]  UdiffTsProdOutMax=[]  NTsProdOutMin=[]  NTsProdOutMax=[]  UintegralTsProdOutMin=[]  UintegralTsProdOutMax=[]  UngainTsProdOutMin=[]  UngainTsProdOutMax=[]  IntegratorContinuousStateAttributes=''  IntegratorStateMustResolveToSignalObject=off  IntegratorRTWStateStorageClass=Auto  FilterContinuousStateAttributes=''  FilterStateMustResolveToSignalObject=off  FilterRTWStateStorageClass=Auto  ParallelPVariant=InternalParameters  IdealPVariant=Disabled  IVariant=InternalParameters  DVariant=InternalParameters  IntegratorVariant=Discrete  SatVariant=Disabled  AWVariant=Passthrough  PCopyVariant=Disabled  TRVariant=Disabled  FdbkBlocksVariant=Forward  IdealPFdbkVariant=Disabled  SatFdbkVariant=Disabled  DerivativeFilterVariant=ForwardEulerFilter  NVariant=InternalParameters  NCopyVariant=Disabled  FilterICVariant=InternalICsFilter  IntegratorICVariant=InternalICs  ExternalResetVariant=Disabled  TRSumVariant=Passthrough  SumFdbkVariant=Disabled  SumVariant=Sum_PID  TsampFilterVariant=InternalTs  TsampNgainVariant=Passthrough  TsampIntegralVariant=Passthrough  ExternalSaturationOutDataTypeStr=Inherit: Same as second input
  cfblk4 : Trigonometry
  cfblk2 : Outport
  wires:
  cfblk4/1 -> cfblk2/1
  cfblk1/1 -> cfblk3/1
  cfblk3/1 -> cfblk4/1

== system sampleModel208/cfblk95 ==
  cfblk1 : Inport
  Action Port : ActionPort  ActionPortLabel=else
  cfblk3 : Sqrt  SaturateOnIntegerOverflow=on
  cfblk2 : Outport
  wires:
  cfblk1/1 -> cfblk2/1, cfblk3/1

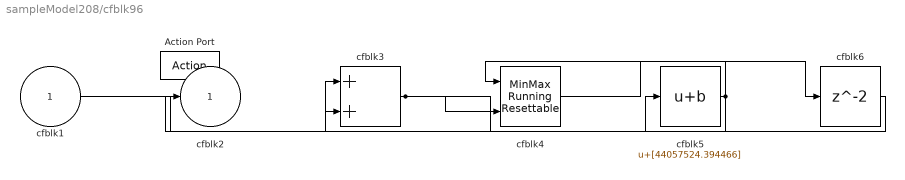
== system sampleModel208/cfblk96 ==
  cfblk1 : Inport
  Action Port : ActionPort  ActionPortLabel=if(u1 >= 0)
  cfblk3 : Sum
  cfblk4 : simulink/Math Operations/MinMax Running Resettable  Function=min  vinit=0.0
  cfblk5 : Bias  Bias=[44057524.394466]
  cfblk6 : Delay
  cfblk2 : Outport
  wires:
  cfblk5/1 -> cfblk4/1, cfblk2/1
  cfblk1/1 -> cfblk3/1
  cfblk3/1 -> cfblk5/1, cfblk4/2
  cfblk4/1 -> cfblk6/1
  cfblk6/1 -> cfblk3/2

== system sampleModel208/cfblk97 ==
  cfblk1 : Inport
  cfblk4 : Inport  Port=2
  Action Port : ActionPort  ActionPortLabel=else
  cfblk3 : ComplexToRealImag
  cfblk2 : Outport
  wires:
  cfblk1/1 -> cfblk2/1
  cfblk4/1 -> cfblk3/1

== system sampleModel208/cfblk98 ==
  cfblk1 : Inport
  Action Port : ActionPort  ActionPortLabel=if(u1 >= 0)
  cfblk3 : Assignment  DiagnosticForDimensions=Warning  IndexOptions=Index vector (dialog)  Indices=1  OutputSizes=1
  cfblk4 : Rounding
  cfblk2 : Outport
  wires:
  cfblk1/1 -> cfblk4/1, cfblk3/2
  cfblk4/1 -> cfblk3/1
  cfblk3/1 -> cfblk2/1

== system sampleModel208/cfblk99 ==
  cfblk1 : Inport
  Action Port : ActionPort  ActionPortLabel=else
  cfblk3 : Sum  Inputs=|++
  cfblk2 : Outport
  wires:
  cfblk1/1 -> cfblk3/1, cfblk3/2
  cfblk3/1 -> cfblk2/1
